simulink model "CompensationTotale"  (R2017a)
settings: Solver=VariableStepAuto  StartTime=0.0  StopTime=10.0  RelTol=1e-3
settings Model: Creator=PC  LastModifiedBy=PC

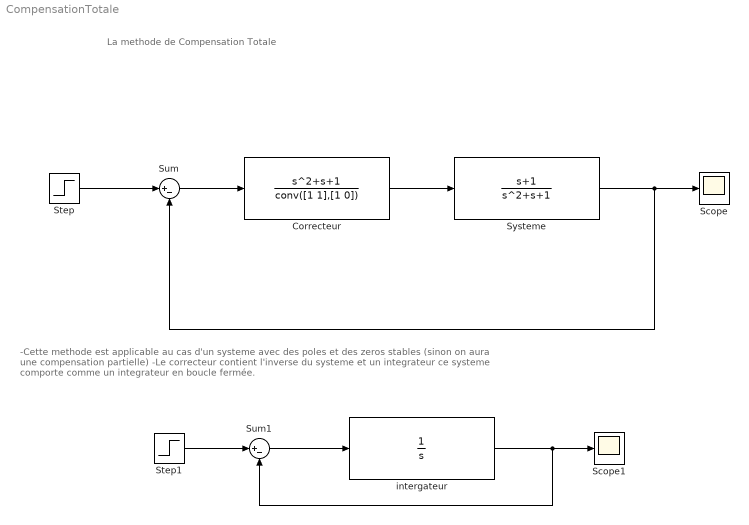
== system CompensationTotale ==
  note: -Cette methode est applicable au cas d'un systeme avec des poles et des zeros stables (sinon on aura une compensation partielle)
      | -Le correcteur contient l'inverse du systeme et un integrateur
      | ce systeme comporte comme un integrateur en boucle fermée.
  note: La methode de Compensation Totale
  Correcteur : TransferFcn  Numerator=[1 1 1]  Denominator=conv([1 1],[1 0])
  Scope : Scope
  Scope1 : Scope
  Step : Step  Time=0  SampleTime=0
  Step1 : Step  Time=0  SampleTime=0
  Sum : Sum  Inputs=|+-
  Sum1 : Sum  Inputs=|+-
  "Systeme " : TransferFcn  Numerator=[1 1]  Denominator=[1 1 1]
  intergateur : TransferFcn  Numerator=1  Denominator=[1 0]
  wires:
  Step/1 -> Sum/1
  Sum/1 -> Correcteur/1
  Correcteur/1 -> "Systeme "/1
  "Systeme "/1 -> Sum/2, Scope/1
  Step1/1 -> Sum1/1
  Sum1/1 -> intergateur/1
  intergateur/1 -> Sum1/2, Scope1/1
